simulink model "Model_Sim_of_State_deviation_FB_PD"  (R2023b)
settings: Solver=ode4  StartTime=0.0  StopTime=Sim_time  FixedStep=Sampling_time  RelTol=1e-3
values from neighbouring files (symbols this model uses):
  Amplitude = 10    [SET_Sim_of_State_deviation_FB_PD.m]    (also in SET_Sim_of_State_deviation_FB_P_D.m; SET_Sim_of_integral_servo_I_PD.m; SET_Sim_of_state_deviation_FB_and_output_integral_PID.m; SET_Sim_of_state_deviation_FB_and_output_integral_PI_D.m)
  Angular_frequency = (2*pi)/Vibration_period    (= 1.57079632679)    [SET_Sim_of_State_deviation_FB_PD.m]    (also in SET_Sim_of_State_deviation_FB_P_D.m; SET_Sim_of_integral_servo_I_PD.m; SET_Sim_of_state_deviation_FB_and_output_integral_PID.m; SET_Sim_of_state_deviation_FB_and_output_integral_PI_D.m)
  c = 1    [Primary system response time.m]    (also in Primary_system_response_time.m; SET_Sim_of_State_deviation_FB_PD.m = 2; SET_Sim_of_State_deviation_FB_P_D.m = 2; SET_Sim_of_integral_servo_I_PD.m = 2)
  Initial_phase = 0    [SET_Sim_of_State_deviation_FB_PD.m]    (also in SET_Sim_of_State_deviation_FB_P_D.m; SET_Sim_of_integral_servo_I_PD.m; SET_Sim_of_state_deviation_FB_and_output_integral_PID.m; SET_Sim_of_state_deviation_FB_and_output_integral_PI_D.m)
  k = 1    [SET_Sim_of_State_deviation_FB_PD.m]    (also in SET_Sim_of_State_deviation_FB_P_D.m; SET_Sim_of_integral_servo_I_PD.m; SET_Sim_of_regulator_control.m; SET_Sim_of_state_deviation_FB_and_output_integral_PID.m)
  Ke = -lqr(A,B,Q,R)    [SET_Sim_of_State_deviation_FB_PD.m]    (also in SET_Sim_of_State_deviation_FB_P_D.m; SET_Sim_of_integral_servo_I_PD.m = tildeKe(:,1:n); SET_Sim_of_state_deviation_FB_and_output_integral_PID.m = tildeKe(:,1:n); SET_Sim_of_state_deviation_FB_and_output_integral_PI_D.m = tildeKe(:,1:n))
  m = 1    [SET_Sim_of_State_deviation_FB_PD.m]    (also in SET_Sim_of_State_deviation_FB_P_D.m; SET_Sim_of_integral_servo_I_PD.m; SET_Sim_of_regulator_control.m; SET_Sim_of_state_deviation_FB_and_output_integral_PID.m)
  Noise_rise_time = 5    [SET_Sim_of_State_deviation_FB_PD.m]    (also in SET_Sim_of_State_deviation_FB_P_D.m; SET_Sim_of_integral_servo_I_PD.m; SET_Sim_of_state_deviation_FB_and_output_integral_PID.m; SET_Sim_of_state_deviation_FB_and_output_integral_PI_D.m)
  Sampling_time = 0.001    [SET_Sim_of_State_deviation_FB_PD.m]    (also in SET_Sim_of_State_deviation_FB_P_D.m; SET_Sim_of_integral_servo_I_PD.m; SET_Sim_of_regulator_control.m; SET_Sim_of_state_deviation_FB_and_output_integral_PID.m)
  Step_noise = -10    [SET_Sim_of_State_deviation_FB_PD.m]    (also in SET_Sim_of_State_deviation_FB_P_D.m; SET_Sim_of_integral_servo_I_PD.m; SET_Sim_of_state_deviation_FB_and_output_integral_PID.m; SET_Sim_of_state_deviation_FB_and_output_integral_PI_D.m)
  Target_angular_frequency = pi/(2*Tfin)    (= 1.57079632679)    [SET_Sim_of_State_deviation_FB_PD.m]    (also in SET_Sim_of_State_deviation_FB_P_D.m; SET_Sim_of_integral_servo_I_PD.m; SET_Sim_of_state_deviation_FB_and_output_integral_PID.m; SET_Sim_of_state_deviation_FB_and_output_integral_PI_D.m)
  Target_value = 10    [SET_Sim_of_State_deviation_FB_PD.m]    (also in SET_Sim_of_State_deviation_FB_P_D.m; SET_Sim_of_integral_servo_I_PD.m; SET_Sim_of_state_deviation_FB_and_output_integral_PID.m; SET_Sim_of_state_deviation_FB_and_output_integral_PI_D.m)
  Tfin = 1    [SET_Sim_of_State_deviation_FB_PD.m]    (also in SET_Sim_of_State_deviation_FB_P_D.m; SET_Sim_of_integral_servo_I_PD.m; SET_Sim_of_state_deviation_FB_and_output_integral_PID.m; SET_Sim_of_state_deviation_FB_and_output_integral_PI_D.m)
  x0 = q0    [Primary system response time.m]    (also in Primary_system_response_time.m; SET_Sim_of_State_deviation_FB_PD.m = zeros(2,1); SET_Sim_of_State_deviation_FB_P_D.m = zeros(2,1); SET_Sim_of_integral_servo_I_PD.m = zeros(2,1))
settings Model: Creator=yuyas  LastModifiedBy=yuyas
settings DataIOCC: ReturnWorkspaceOutputs=off

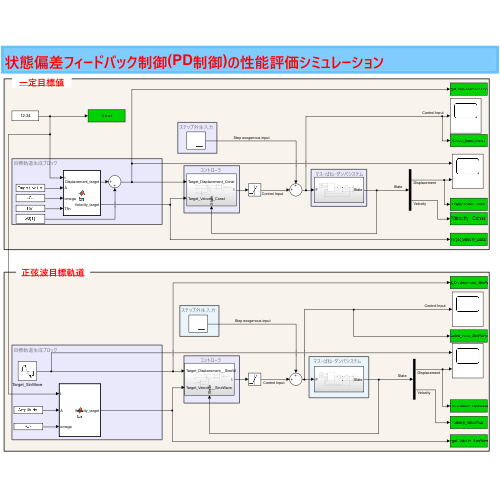
[thumbnail: Simulink's stored preview of the top-level diagram]
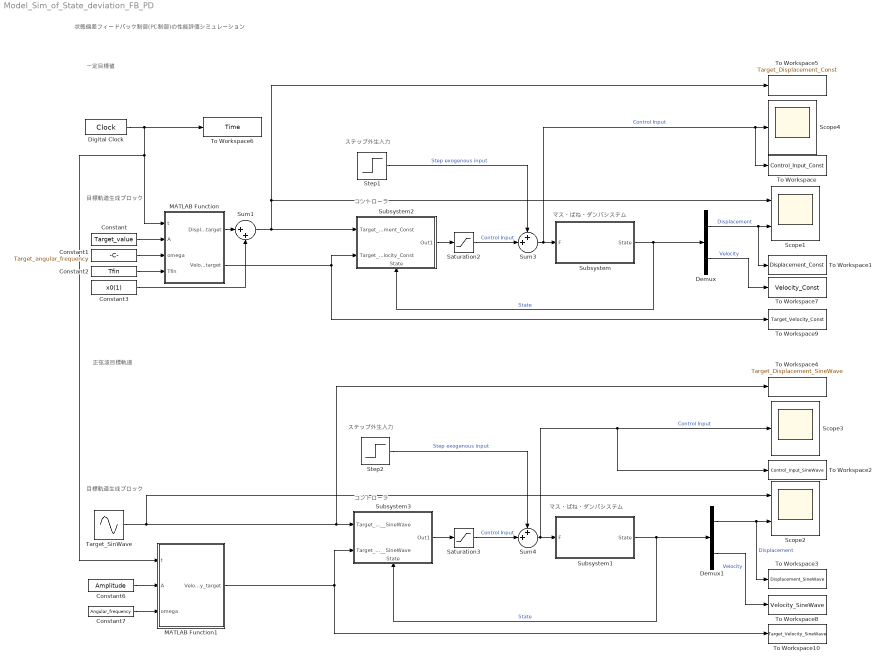
== system Model_Sim_of_State_deviation_FB_PD ==
  note: 目標軌道生成ブロック
  note: 状態偏差フィードバック制御(PD制御)の性能評価シミュレーション
  note: ステップ外生入力
  note: マス・ばね・ダンパシステム
  note: 一定目標値
  note: マス・ばね・ダンパシステム
  note: 正弦波目標軌道
  note: ステップ外生入力
  note: コントローラ
  note: 目標軌道生成ブロック
  note: コントローラ
  Constant : Constant  Value=Target_value
  Constant1 : Constant  Value=Target_angular_frequency
  Constant2 : Constant  Value=Tfin
  Constant3 : Constant  Value=x0(1)
  Constant6 : Constant  Value=Amplitude
  Constant7 : Constant  Value=Angular_frequency
  Demux : Demux  Outputs=2
  Demux1 : Demux  Outputs=2
  Digital Clock : DigitalClock  SampleTime=Sampling_time
  MATLAB Function : MATLAB Function  TreatAsAtomicUnit=on
  MATLAB Function1 : MATLAB Function  TreatAsAtomicUnit=on
  Saturation2 : Saturate  UpperLimit=200  LowerLimit=-200
  Saturation3 : Saturate  UpperLimit=200  LowerLimit=-200
  Scope1 : Scope  NumInputPorts=2
  Scope2 : Scope  NumInputPorts=2
  Scope3 : Scope
  Scope4 : Scope
  Step1 : Step  Time=Noise_rise_time  After=Step_noise  SampleTime=0
  Step2 : Step  Time=Noise_rise_time  After=Step_noise  SampleTime=0
  Subsystem : Subsystem
  Subsystem1 : Subsystem
  Subsystem2 : Subsystem
      settings: PortSchema="{\"entries\":[{\"content\":{\"sides\":[{\"content\":{\"connectorIds\":[\"In1\",\"In2\"]},\"type\":\"ConnectorPlacement.EquallySpacedRectSide\",\"uuid\":\"008c5a85-5064-422e-8dea-11f1134d59bc\"},{\"content\":{\"connectorIds\":[\"Out1\"],\"side\":\"RIGHT\"},\"type\":\"ConnectorPlacement.EquallySpacedRectSide\",\"uuid\":\"19bc85aa-318c-4dd8-8798-b61a9a5fb079\"},{\"content\":{\"side\":\"TOP\"},\"type\":\"ConnectorPlacement.EquallySpacedRectSide\",\"uuid\":\"eddf1bb5-9d97-4ef5-9025-aea1a50b7a07\"},{\"content\":{\"connectorIds\":[\"In3\"],\"side\":\"BOTTOM\"},\"type\":\"ConnectorPlacement.EquallySpacedRectSide\",\"uuid\":\"f998d74c-636c-474d-835b-000fc1bfc6a3\"}]},\"type\":\"ConnectorPlacement.EquallySpacedConnector\",\"uuid\":\"4fcfd2d1-f977-49d4-b23c-2c722631ea93\"}],\"packageUris\":[\"http://schema.mathworks.com/mf0/Connector/R2020b\"],\"version\":\"1.0\"}"
  Subsystem3 : Subsystem
      settings: PortSchema="{\"entries\":[{\"content\":{\"sides\":[{\"content\":{\"connectorIds\":[\"In1\",\"In2\"]},\"type\":\"ConnectorPlacement.EquallySpacedRectSide\",\"uuid\":\"008c5a85-5064-422e-8dea-11f1134d59bc\"},{\"content\":{\"connectorIds\":[\"Out1\"],\"side\":\"RIGHT\"},\"type\":\"ConnectorPlacement.EquallySpacedRectSide\",\"uuid\":\"19bc85aa-318c-4dd8-8798-b61a9a5fb079\"},{\"content\":{\"side\":\"TOP\"},\"type\":\"ConnectorPlacement.EquallySpacedRectSide\",\"uuid\":\"eddf1bb5-9d97-4ef5-9025-aea1a50b7a07\"},{\"content\":{\"connectorIds\":[\"In3\"],\"side\":\"BOTTOM\"},\"type\":\"ConnectorPlacement.EquallySpacedRectSide\",\"uuid\":\"f998d74c-636c-474d-835b-000fc1bfc6a3\"}]},\"type\":\"ConnectorPlacement.EquallySpacedConnector\",\"uuid\":\"4fcfd2d1-f977-49d4-b23c-2c722631ea93\"}],\"packageUris\":[\"http://schema.mathworks.com/mf0/Connector/R2020b\"],\"version\":\"1.0\"}"
  Sum1 : Sum  Inputs=|++
  Sum3 : Sum  Inputs=++|
  Sum4 : Sum  Inputs=++|
  Target_SinWave : Sin  Amplitude=Amplitude  Frequency=Angular_frequency  Phase=Initial_phase  SampleTime=Sampling_time  VectorParams1D=off
  To Workspace : ToWorkspace  VariableName=Control_Input_Const  SampleTime=-1
      settings: Save2DSignal=2-D array (concatenate along first dimension)
  To Workspace1 : ToWorkspace  VariableName=Displacement_Const  SampleTime=-1
      settings: Save2DSignal=2-D array (concatenate along first dimension)
  To Workspace10 : ToWorkspace  VariableName=Target_Velocity_SineWave  SampleTime=-1
      settings: Save2DSignal=2-D array (concatenate along first dimension)
  To Workspace2 : ToWorkspace  VariableName=Control_Input_SineWave  SampleTime=-1
      settings: Save2DSignal=2-D array (concatenate along first dimension)
  To Workspace3 : ToWorkspace  VariableName=Displacement_SineWave  SampleTime=-1
      settings: Save2DSignal=2-D array (concatenate along first dimension)
  To Workspace4 : ToWorkspace  VariableName=Target_Displacement_SineWave  SampleTime=-1
      settings: Save2DSignal=2-D array (concatenate along first dimension)
  To Workspace5 : ToWorkspace  VariableName=Target_Displacement_Const  SampleTime=-1
      settings: Save2DSignal=2-D array (concatenate along first dimension)
  To Workspace6 : ToWorkspace  VariableName=Time  SampleTime=-1
      settings: Save2DSignal=2-D array (concatenate along first dimension)
  To Workspace7 : ToWorkspace  VariableName=Velocity_Const  SampleTime=-1
      settings: Save2DSignal=2-D array (concatenate along first dimension)
  To Workspace8 : ToWorkspace  VariableName=Velocity_SineWave  SampleTime=-1
      settings: Save2DSignal=2-D array (concatenate along first dimension)
  To Workspace9 : ToWorkspace  VariableName=Target_Velocity_Const  SampleTime=-1
      settings: Save2DSignal=2-D array (concatenate along first dimension)
  wires:
  Sum3/1 -> To Workspace/1, Scope4/1, Subsystem/1(F)  "Control Input"
  Step1/1 -> Sum3/1  "Step exogenous input"
  Subsystem/1(State) -> Demux/1, Subsystem2/3(State)  "State"
  Demux/2 -> To Workspace7/1  "Velocity"
  Demux/1 -> To Workspace1/1, Scope1/2  "Displacement"
  Demux1/1 -> To Workspace3/1, Scope2/2  "Displacement"
  Sum4/1 -> To Workspace2/1, Scope3/1, Subsystem1/1(F)  "Control Input"
  Demux1/2 -> To Workspace8/1  "Velocity"
  Step2/1 -> Sum4/1  "Step exogenous input"
  Digital Clock/1 -> MATLAB Function1/1(t), MATLAB Function/1(t), To Workspace6/1
  Subsystem2/1(Out1) -> Saturation2/1
  Target_SinWave/1 -> Scope2/1, To Workspace4/1, Subsystem3/1(Target_Displacement__SineWave)
  Subsystem1/1(State) -> Demux1/1, Subsystem3/3(State)  "State"
  Subsystem3/1(Out1) -> Saturation3/1
  Saturation2/1 -> Sum3/2  "Control Input"
  Saturation3/1 -> Sum4/2  "Control Input"
  Constant/1 -> MATLAB Function/2(A)
  Constant1/1 -> MATLAB Function/3(omega)
  Constant2/1 -> MATLAB Function/4(Tfin)
  MATLAB Function/1(Displacement_target) -> Sum1/1
  Constant3/1 -> Sum1/2
  Sum1/1 -> Subsystem2/1(Target_Displacement_Const), Scope1/1, To Workspace5/1
  MATLAB Function1/1(Velocity_target) -> To Workspace10/1, Subsystem3/2(Target_Velocity__SineWave)
  Constant7/1 -> MATLAB Function1/3(omega)
  Constant6/1 -> MATLAB Function1/2(A)
  MATLAB Function/2(Velocity_target) -> To Workspace9/1, Subsystem2/2(Target_Velocity_Const)

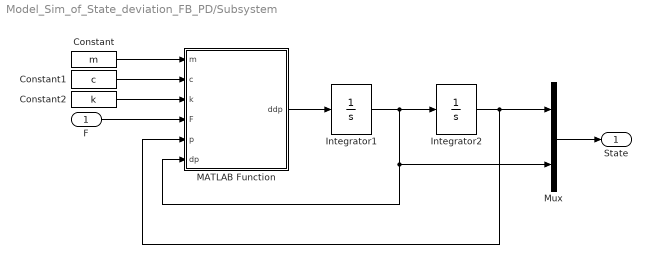
== system Model_Sim_of_State_deviation_FB_PD/Subsystem ==
  F : Inport
  Constant : Constant  Value=m
  Constant1 : Constant  Value=c
  Constant2 : Constant  Value=k
  Integrator1 : Integrator  InitialCondition=x0(2,1)
  Integrator2 : Integrator  InitialCondition=x0(1,1)
  MATLAB Function : MATLAB Function  TreatAsAtomicUnit=on
  Mux : Mux  Inputs=2
  State : Outport  PortDimensions=2
  wires:
  MATLAB Function/1(ddp) -> Integrator1/1
  F/1 -> MATLAB Function/4(F)
  Integrator1/1 -> Integrator2/1, MATLAB Function/6(dp), Mux/2
  Integrator2/1 -> MATLAB Function/5(p), Mux/1
  Mux/1 -> State/1
  Constant/1 -> MATLAB Function/1(m)
  Constant1/1 -> MATLAB Function/2(c)
  Constant2/1 -> MATLAB Function/3(k)

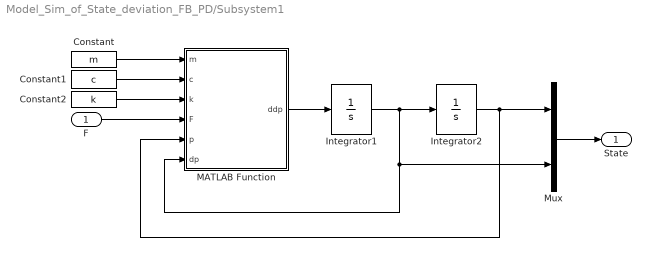
== system Model_Sim_of_State_deviation_FB_PD/Subsystem1 ==
  F : Inport
  Constant : Constant  Value=m
  Constant1 : Constant  Value=c
  Constant2 : Constant  Value=k
  Integrator1 : Integrator  InitialCondition=x0(1,1)
  Integrator2 : Integrator  InitialCondition=x0(2,1)
  MATLAB Function : MATLAB Function  TreatAsAtomicUnit=on
  Mux : Mux  Inputs=2
  State : Outport  PortDimensions=2
  wires:
  MATLAB Function/1(ddp) -> Integrator1/1
  F/1 -> MATLAB Function/4(F)
  Integrator1/1 -> Integrator2/1, MATLAB Function/6(dp), Mux/2
  Integrator2/1 -> MATLAB Function/5(p), Mux/1
  Mux/1 -> State/1
  Constant/1 -> MATLAB Function/1(m)
  Constant1/1 -> MATLAB Function/2(c)
  Constant2/1 -> MATLAB Function/3(k)

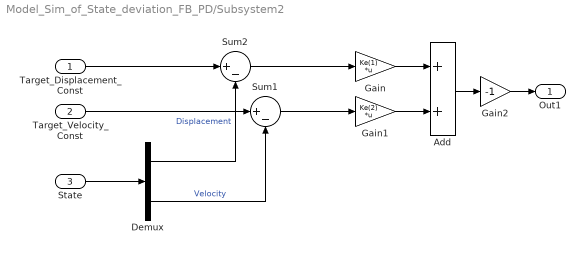
== system Model_Sim_of_State_deviation_FB_PD/Subsystem2 ==
  Target_Displacement_Const : Inport
  Target_Velocity_Const : Inport  Port=2
  State : Inport  Port=3
  Add : Sum
  Demux : Demux  Outputs=2
  Gain : Gain  Gain=Ke(1)  Multiplication=Matrix(K*u)
  Gain1 : Gain  Gain=Ke(2)  Multiplication=Matrix(K*u)
  Gain2 : Gain  Gain=-1
  Sum1 : Sum  Inputs=|+-
  Sum2 : Sum  Inputs=|+-
  Out1 : Outport
  wires:
  Target_Displacement_Const/1 -> Sum2/1
  State/1 -> Demux/1
  Demux/1 -> Sum2/2  "Displacement"
  Target_Velocity_Const/1 -> Sum1/1
  Demux/2 -> Sum1/2  "Velocity"
  Sum2/1 -> Gain/1
  Sum1/1 -> Gain1/1
  Gain/1 -> Add/1
  Gain1/1 -> Add/2
  Add/1 -> Gain2/1
  Gain2/1 -> Out1/1

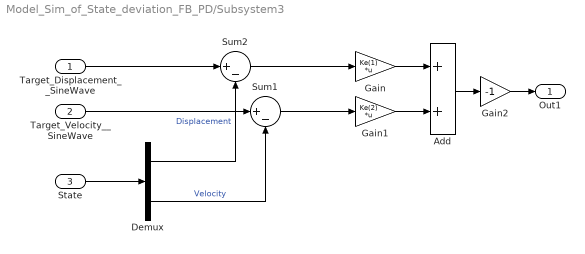
== system Model_Sim_of_State_deviation_FB_PD/Subsystem3 ==
  Target_Displacement__SineWave : Inport
  Target_Velocity__SineWave : Inport  Port=2
  State : Inport  Port=3
  Add : Sum
  Demux : Demux  Outputs=2
  Gain : Gain  Gain=Ke(1)  Multiplication=Matrix(K*u)
  Gain1 : Gain  Gain=Ke(2)  Multiplication=Matrix(K*u)
  Gain2 : Gain  Gain=-1
  Sum1 : Sum  Inputs=|+-
  Sum2 : Sum  Inputs=|+-
  Out1 : Outport
  wires:
  Target_Displacement__SineWave/1 -> Sum2/1
  State/1 -> Demux/1
  Demux/1 -> Sum2/2  "Displacement"
  Target_Velocity__SineWave/1 -> Sum1/1
  Demux/2 -> Sum1/2  "Velocity"
  Sum2/1 -> Gain/1
  Sum1/1 -> Gain1/1
  Gain/1 -> Add/1
  Gain1/1 -> Add/2
  Add/1 -> Gain2/1
  Gain2/1 -> Out1/1

== matlab function Model_Sim_of_State_deviation_FB_PD/Subsystem1/MATLAB Function ==
  data: m input; c input; k input; F input; ddp output; p input; dp input
function ddp = fcn(m, c, k, F,p,dp)

ddp = (-c/m)*dp+(-c/m)*p+(1/m)*F;

end

== matlab function Model_Sim_of_State_deviation_FB_PD/Subsystem/MATLAB Function ==
  data: m input; c input; k input; F input; ddp output; p input; dp input
function ddp = fcn(m, c, k, F,p,dp)

ddp = (-c/m)*dp+(-c/m)*p+(1/m)*F;

end

== matlab function Model_Sim_of_State_deviation_FB_PD/MATLAB Function ==
  data: t input; A input; Displacement_target output; omega input; Tfin input; Velocity_target output
function [Displacement_target, Velocity_target]= fcn(t,A,omega,Tfin)
if (t >= Tfin)
    Displacement_target = A;
    Velocity_target = 0;
else
    Displacement_target = A * (1-cos(omega*t));
    Velocity_target = omega * A * sin(omega * t);
end

== matlab function Model_Sim_of_State_deviation_FB_PD/MATLAB Function1 ==
  data: t input; A input; omega input; Velocity_target output
function Velocity_target = fcn(t,A,omega)
     Velocity_target = A * omega * cos(omega * t);
end
